simulink model "move_to_pose_R2020a1"  (R2020a)
settings: Solver=FixedStepAuto  StartTime=0.0  StopTime=inf  FixedStep=sampleTime  RelTol=1e-3
PreLoadFcn:
  | % Simulation parameters
  | load exampleMap
  | sampleTime = 0.05;
  | 
  | % Robot parameters
  | wheelRadius = 0.05;
  | robotRadius = 0.5;
  | 
  | % Lidar parameters
  | sensorOffset = [0,0];
  | scanAngles = linspace(-pi/2,pi/2,9)';
  | maxRange = 25;
undefined symbols (not defined in the file or in its folder): data_array
libraries: mobileRoboticsLib x38, robotalgslib x11, mobileRoboticsTrainingLib x11
settings Model: SimulationMode=accelerator  EnablePacing=on  PacingRate=1000  Creator=scastro  LastModifiedBy=prans
settings DataIOCC: ReturnWorkspaceOutputs=off
settings DebuggingCC: PregeneratedLibrarySubsystemCodeDiagnostic=none  ArithmeticOperatorsInVariantConditions=warning
settings SFSimCC: SimUseLocalCustomCode=off  CustomCodeUndefinedFunction=UseInterfaceOnly
settings RTWCC: RTWUseLocalCustomCode=off

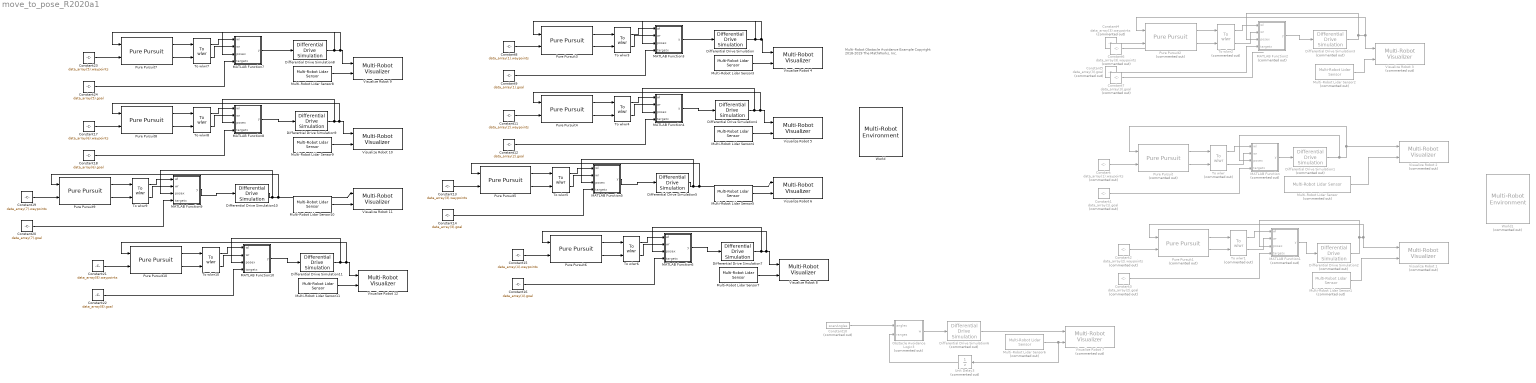
== system move_to_pose_R2020a1 ==
  note: Multi-Robot Obstacle
      | Avoidance Example
      |
      | Copyright 2018-2019 The MathWorks, Inc.
  Constant : Constant  Commented=on  Value=data_array(1).waypoints
  Constant1 : Constant  Commented=on  Value=data_array(1).goal
  Constant10 : Constant  Commented=on  Value=scanAngles
  Constant11 : Constant  Value=data_array(2).waypoints
  Constant12 : Constant  Value=data_array(2).goal
  Constant13 : Constant  Value=data_array(3).waypoints
  Constant14 : Constant  Value=data_array(3).goal
  Constant15 : Constant  Value=data_array(4).waypoints
  Constant16 : Constant  Value=data_array(4).goal
  Constant17 : Constant  Value=data_array(6).waypoints
  Constant18 : Constant  Value=data_array(6).goal
  Constant19 : Constant  Value=data_array(7).waypoints
  Constant2 : Constant  Commented=on  Value=data_array(2).waypoints
  Constant20 : Constant  Value=data_array(7).goal
  Constant21 : Constant  Value=data_array(8).waypoints
  Constant22 : Constant  Value=data_array(8).goal
  Constant23 : Constant  Value=data_array(5).waypoints
  Constant24 : Constant  Value=data_array(5).goal
  Constant3 : Constant  Commented=on  Value=data_array(2).goal
  Constant4 : Constant  Commented=on  Value=data_array(3).waypoints
  Constant5 : Constant  Commented=on  Value=data_array(3).goal
  Constant6 : Constant  Commented=on  Value=data_array(3).waypoints
  Constant7 : Constant  Commented=on  Value=data_array(3).goal
  Constant8 : Constant  Value=data_array(1).waypoints
  Constant9 : Constant  Value=data_array(1).goal
  Differential Drive Simulation : mobileRoboticsLib/Kinematic Models/Differential Drive/Differential Drive Simulation  wheelRadius=wheelRadius  wheelBase=robotRadius  initX=data_array(1).start(1)  initY=data_array(1).start(2)  initAngle=0  Ts=sampleTime
      settings: SourceProductName=Mobile Robotics Simulation Toolbox
  Differential Drive Simulation1 : mobileRoboticsLib/Kinematic Models/Differential Drive/Differential Drive Simulation  Commented=on  wheelRadius=wheelRadius  wheelBase=robotRadius  initX=data_array(1).start(1)  initY=data_array(1).start(2)  initAngle=0  Ts=sampleTime
      settings: SourceProductName=Mobile Robotics Simulation Toolbox
  Differential Drive Simulation10 : mobileRoboticsLib/Kinematic Models/Differential Drive/Differential Drive Simulation  wheelRadius=wheelRadius  wheelBase=robotRadius  initX=data_array(7).start(1)  initY=data_array(7).start(2)  initAngle=-pi/4  Ts=sampleTime
      settings: SourceProductName=Mobile Robotics Simulation Toolbox
  Differential Drive Simulation11 : mobileRoboticsLib/Kinematic Models/Differential Drive/Differential Drive Simulation  wheelRadius=wheelRadius  wheelBase=robotRadius  initX=data_array(8).start(1)  initY=data_array(8).start(2)  initAngle=-pi/4  Ts=sampleTime
      settings: SourceProductName=Mobile Robotics Simulation Toolbox
  Differential Drive Simulation2 : mobileRoboticsLib/Kinematic Models/Differential Drive/Differential Drive Simulation  Commented=on  wheelRadius=wheelRadius  wheelBase=robotRadius  initX=data_array(2).start(1)  initY=data_array(2).start(2)  initAngle=pi/2  Ts=sampleTime
      settings: SourceProductName=Mobile Robotics Simulation Toolbox
  Differential Drive Simulation3 : mobileRoboticsLib/Kinematic Models/Differential Drive/Differential Drive Simulation  Commented=on  wheelRadius=wheelRadius  wheelBase=robotRadius  initX=data_array(3).start(1)  initY=data_array(3).start(2)  initAngle=-pi/4  Ts=sampleTime
      settings: SourceProductName=Mobile Robotics Simulation Toolbox
  Differential Drive Simulation4 : mobileRoboticsLib/Kinematic Models/Differential Drive/Differential Drive Simulation  wheelRadius=wheelRadius  wheelBase=robotRadius  initX=data_array(2).start(1)  initY=data_array(2).start(2)  initAngle=pi/2  Ts=sampleTime
      settings: SourceProductName=Mobile Robotics Simulation Toolbox
  Differential Drive Simulation5 : mobileRoboticsLib/Kinematic Models/Differential Drive/Differential Drive Simulation  wheelRadius=wheelRadius  wheelBase=robotRadius  initX=data_array(3).start(1)  initY=data_array(3).start(2)  initAngle=-pi/4  Ts=sampleTime
      settings: SourceProductName=Mobile Robotics Simulation Toolbox
  Differential Drive Simulation6 : mobileRoboticsLib/Kinematic Models/Differential Drive/Differential Drive Simulation  Commented=on  wheelRadius=wheelRadius  wheelBase=robotRadius  initX=8  initY=8  initAngle=-pi/4  Ts=sampleTime
      settings: SourceProductName=Mobile Robotics Simulation Toolbox
  Differential Drive Simulation7 : mobileRoboticsLib/Kinematic Models/Differential Drive/Differential Drive Simulation  wheelRadius=wheelRadius  wheelBase=robotRadius  initX=data_array(4).start(1)  initY=data_array(4).start(2)  initAngle=-pi/4  Ts=sampleTime
      settings: SourceProductName=Mobile Robotics Simulation Toolbox
  Differential Drive Simulation8 : mobileRoboticsLib/Kinematic Models/Differential Drive/Differential Drive Simulation  wheelRadius=wheelRadius  wheelBase=robotRadius  initX=data_array(5).start(1)  initY=data_array(5).start(2)  initAngle=0  Ts=sampleTime
      settings: SourceProductName=Mobile Robotics Simulation Toolbox
  Differential Drive Simulation9 : mobileRoboticsLib/Kinematic Models/Differential Drive/Differential Drive Simulation  wheelRadius=wheelRadius  wheelBase=robotRadius  initX=data_array(6).start(1)  initY=data_array(6).start(2)  initAngle=pi/2  Ts=sampleTime
      settings: SourceProductName=Mobile Robotics Simulation Toolbox
  MATLAB Function : MATLAB Function  Commented=on  TreatAsAtomicUnit=on
  MATLAB Function1 : MATLAB Function  Commented=on  TreatAsAtomicUnit=on
  MATLAB Function10 : MATLAB Function  TreatAsAtomicUnit=on
  MATLAB Function2 : MATLAB Function  Commented=on  TreatAsAtomicUnit=on
  MATLAB Function3 : MATLAB Function  TreatAsAtomicUnit=on
  MATLAB Function4 : MATLAB Function  TreatAsAtomicUnit=on
  MATLAB Function5 : MATLAB Function  TreatAsAtomicUnit=on
  MATLAB Function6 : MATLAB Function  TreatAsAtomicUnit=on
  MATLAB Function7 : MATLAB Function  TreatAsAtomicUnit=on
  MATLAB Function8 : MATLAB Function  TreatAsAtomicUnit=on
  MATLAB Function9 : MATLAB Function  TreatAsAtomicUnit=on
  Multi-Robot Lidar Sensor : mobileRoboticsLib/Environments/Multi-Robot Lidar Sensor  Commented=on  robotIdx=1  mapName=map  sensorOffset=sensorOffset  scanAngles=scanAngles  maxRange=maxRange
      settings: SourceProductName=Mobile Robotics Simulation Toolbox
  Multi-Robot Lidar Sensor1 : mobileRoboticsLib/Environments/Multi-Robot Lidar Sensor  Commented=on  robotIdx=2  mapName=map  sensorOffset=sensorOffset  scanAngles=scanAngles  maxRange=maxRange
      settings: SourceProductName=Mobile Robotics Simulation Toolbox
  Multi-Robot Lidar Sensor10 : mobileRoboticsLib/Environments/Multi-Robot Lidar Sensor  robotIdx=7  mapName=map  sensorOffset=sensorOffset  scanAngles=scanAngles  maxRange=maxRange
      settings: SourceProductName=Mobile Robotics Simulation Toolbox
  Multi-Robot Lidar Sensor11 : mobileRoboticsLib/Environments/Multi-Robot Lidar Sensor  robotIdx=8  mapName=map  sensorOffset=sensorOffset  scanAngles=scanAngles  maxRange=maxRange
      settings: SourceProductName=Mobile Robotics Simulation Toolbox
  Multi-Robot Lidar Sensor2 : mobileRoboticsLib/Environments/Multi-Robot Lidar Sensor  Commented=on  robotIdx=3  mapName=map  sensorOffset=sensorOffset  scanAngles=scanAngles  maxRange=maxRange
      settings: SourceProductName=Mobile Robotics Simulation Toolbox
  Multi-Robot Lidar Sensor3 : mobileRoboticsLib/Environments/Multi-Robot Lidar Sensor  robotIdx=1  mapName=map  sensorOffset=sensorOffset  scanAngles=scanAngles  maxRange=maxRange
      settings: SourceProductName=Mobile Robotics Simulation Toolbox
  Multi-Robot Lidar Sensor4 : mobileRoboticsLib/Environments/Multi-Robot Lidar Sensor  robotIdx=2  mapName=map  sensorOffset=sensorOffset  scanAngles=scanAngles  maxRange=maxRange
      settings: SourceProductName=Mobile Robotics Simulation Toolbox
  Multi-Robot Lidar Sensor5 : mobileRoboticsLib/Environments/Multi-Robot Lidar Sensor  robotIdx=3  mapName=map  sensorOffset=sensorOffset  scanAngles=scanAngles  maxRange=maxRange
      settings: SourceProductName=Mobile Robotics Simulation Toolbox
  Multi-Robot Lidar Sensor6 : mobileRoboticsLib/Environments/Multi-Robot Lidar Sensor  Commented=on  robotIdx=4  mapName=map  sensorOffset=sensorOffset  scanAngles=scanAngles  maxRange=maxRange
      settings: SourceProductName=Mobile Robotics Simulation Toolbox
  Multi-Robot Lidar Sensor7 : mobileRoboticsLib/Environments/Multi-Robot Lidar Sensor  robotIdx=4  mapName=map  sensorOffset=sensorOffset  scanAngles=scanAngles  maxRange=maxRange
      settings: SourceProductName=Mobile Robotics Simulation Toolbox
  Multi-Robot Lidar Sensor8 : mobileRoboticsLib/Environments/Multi-Robot Lidar Sensor  robotIdx=5  mapName=map  sensorOffset=sensorOffset  scanAngles=scanAngles  maxRange=maxRange
      settings: SourceProductName=Mobile Robotics Simulation Toolbox
  Multi-Robot Lidar Sensor9 : mobileRoboticsLib/Environments/Multi-Robot Lidar Sensor  robotIdx=6  mapName=map  sensorOffset=sensorOffset  scanAngles=scanAngles  maxRange=maxRange
      settings: SourceProductName=Mobile Robotics Simulation Toolbox
  Obstacle Avoidance Logic3 : Stateflow chart  Commented=on  TreatAsAtomicUnit=on
  Pure Pursuit : robotalgslib/Pure Pursuit  Commented=on  DesiredLinearVelocity=0.1  MaxAngularVelocity=1  LookaheadDistance=1  TargetDirPort=off  SimulateUsing=Code generation
  Pure Pursuit1 : robotalgslib/Pure Pursuit  Commented=on  DesiredLinearVelocity=0.1  MaxAngularVelocity=1  LookaheadDistance=1  TargetDirPort=off  SimulateUsing=Code generation
  Pure Pursuit{3..10} (8 alike) : robotalgslib/Pure Pursuit  DesiredLinearVelocity=0.1  MaxAngularVelocity=1  LookaheadDistance=1  TargetDirPort=off  SimulateUsing=Code generation
  Pure Pursuit2 : robotalgslib/Pure Pursuit  Commented=on  DesiredLinearVelocity=0.1  MaxAngularVelocity=1  LookaheadDistance=1  TargetDirPort=off  SimulateUsing=Code generation
  To wlwr : mobileRoboticsTrainingLib/To wlwr  Commented=on  axleLength=0.1  wheelR=0.05
  To wlwr1 : mobileRoboticsTrainingLib/To wlwr  Commented=on  axleLength=0.1  wheelR=0.05
  To wlwr{3..10} (8 alike) : mobileRoboticsTrainingLib/To wlwr  axleLength=0.1  wheelR=0.05
  To wlwr2 : mobileRoboticsTrainingLib/To wlwr  Commented=on  axleLength=0.1  wheelR=0.05
  Unit Delay3 : UnitDelay  Commented=on  SampleTime=-1  HasFrameUpgradeWarning=on
  Visualize Robot 1 : mobileRoboticsLib/Environments/Multi-Robot Visualizer  Commented=on  idx=2  radius=robotRadius  robotColor=[0 0 1]  showTraj=off  hasLidar=on  sensorOffset=sensorOffset  scanAngles=scanAngles  maxNumScans=0  hasObjDetector=off  objDetectorOffset=[0 0]  objDetectorAngle=0  objDetectorFOV=pi/2  objDetectorMaxRange=5  hasRobotDetector=off  robotDetectorOffset=[0,0]  robotDetectorAngle=0  robotDetectorFOV=pi/3  robotDetectorMaxRange=5  robotDetectorNumDetections=0
      settings: SourceProductName=Mobile Robotics Simulation Toolbox
  Visualize Robot 10 : mobileRoboticsLib/Environments/Multi-Robot Visualizer  idx=6  radius=robotRadius  robotColor=[1 1 0]  showTraj=on  hasLidar=on  sensorOffset=sensorOffset  scanAngles=scanAngles  maxNumScans=0  hasObjDetector=off  objDetectorOffset=[0 0]  objDetectorAngle=0  objDetectorFOV=pi/2  objDetectorMaxRange=5  hasRobotDetector=off  robotDetectorOffset=[0,0]  robotDetectorAngle=0  robotDetectorFOV=pi/3  robotDetectorMaxRange=5  robotDetectorNumDetections=0
      settings: SourceProductName=Mobile Robotics Simulation Toolbox
  Visualize Robot 11 : mobileRoboticsLib/Environments/Multi-Robot Visualizer  idx=7  radius=robotRadius  robotColor=[1 1 1]  showTraj=on  hasLidar=on  sensorOffset=sensorOffset  scanAngles=scanAngles  maxNumScans=0  hasObjDetector=off  objDetectorOffset=[0 0]  objDetectorAngle=0  objDetectorFOV=pi/2  objDetectorMaxRange=5  hasRobotDetector=off  robotDetectorOffset=[0,0]  robotDetectorAngle=0  robotDetectorFOV=pi/3  robotDetectorMaxRange=5  robotDetectorNumDetections=0
      settings: SourceProductName=Mobile Robotics Simulation Toolbox
  Visualize Robot 12 : mobileRoboticsLib/Environments/Multi-Robot Visualizer  idx=8  radius=robotRadius  robotColor=[0 0 0]  showTraj=on  hasLidar=on  sensorOffset=sensorOffset  scanAngles=scanAngles  maxNumScans=0  hasObjDetector=off  objDetectorOffset=[0 0]  objDetectorAngle=0  objDetectorFOV=pi/2  objDetectorMaxRange=5  hasRobotDetector=off  robotDetectorOffset=[0,0]  robotDetectorAngle=0  robotDetectorFOV=pi/3  robotDetectorMaxRange=5  robotDetectorNumDetections=0
      settings: SourceProductName=Mobile Robotics Simulation Toolbox
  Visualize Robot 2 : mobileRoboticsLib/Environments/Multi-Robot Visualizer  Commented=on  idx=1  radius=robotRadius  robotColor=[1 0 0]  showTraj=off  hasLidar=on  sensorOffset=sensorOffset  scanAngles=scanAngles  maxNumScans=0  hasObjDetector=off  objDetectorOffset=[0,0]  objDetectorAngle=0  objDetectorFOV=pi/2  objDetectorMaxRange=5  hasRobotDetector=off  robotDetectorOffset=sensorOffset  robotDetectorAngle=[pi/2 -pi/2]  robotDetectorFOV=pi  robotDetectorMaxRange=25  robotDetectorNumDetections=0
      link override Goto_ObjDetector: GotoTag=slMultiRobotEnv_ObjDet_2
      link override Goto_Pose: GotoTag=slMultiRobotEnv_Pose_2
      link override Goto_Ranges: GotoTag=slMultiRobotEnv_Ranges_2
      link override Goto_RobotDetector: GotoTag=slMultiRobotEnv_RobotDet_2
      link override Goto_Visuals: GotoTag=slMultiRobotEnv_Visuals_2
      settings: SourceProductName=Mobile Robotics Simulation Toolbox
  Visualize Robot 3 : mobileRoboticsLib/Environments/Multi-Robot Visualizer  Commented=on  idx=3  radius=robotRadius  robotColor=[0 0 1]  showTraj=off  hasLidar=on  sensorOffset=sensorOffset  scanAngles=scanAngles  maxNumScans=0  hasObjDetector=off  objDetectorOffset=[0 0]  objDetectorAngle=0  objDetectorFOV=pi/2  objDetectorMaxRange=5  hasRobotDetector=off  robotDetectorOffset=[0,0]  robotDetectorAngle=0  robotDetectorFOV=pi/3  robotDetectorMaxRange=5  robotDetectorNumDetections=0
      settings: SourceProductName=Mobile Robotics Simulation Toolbox
  Visualize Robot 4 : mobileRoboticsLib/Environments/Multi-Robot Visualizer  idx=1  radius=robotRadius  robotColor=[0 0 1]  showTraj=on  hasLidar=on  sensorOffset=sensorOffset  scanAngles=scanAngles  maxNumScans=0  hasObjDetector=off  objDetectorOffset=[0,0]  objDetectorAngle=0  objDetectorFOV=pi/2  objDetectorMaxRange=5  hasRobotDetector=off  robotDetectorOffset=[0,0]  robotDetectorAngle=0  robotDetectorFOV=pi/3  robotDetectorMaxRange=5  robotDetectorNumDetections=0
      settings: SourceProductName=Mobile Robotics Simulation Toolbox
  Visualize Robot 5 : mobileRoboticsLib/Environments/Multi-Robot Visualizer  idx=2  radius=robotRadius  robotColor=[0 1 0]  showTraj=on  hasLidar=on  sensorOffset=sensorOffset  scanAngles=scanAngles  maxNumScans=0  hasObjDetector=off  objDetectorOffset=[0 0]  objDetectorAngle=0  objDetectorFOV=pi/2  objDetectorMaxRange=5  hasRobotDetector=off  robotDetectorOffset=[0,0]  robotDetectorAngle=0  robotDetectorFOV=pi/3  robotDetectorMaxRange=5  robotDetectorNumDetections=0
      settings: SourceProductName=Mobile Robotics Simulation Toolbox
  Visualize Robot 6 : mobileRoboticsLib/Environments/Multi-Robot Visualizer  idx=3  radius=robotRadius  robotColor=[0 1 1]  showTraj=on  hasLidar=on  sensorOffset=sensorOffset  scanAngles=scanAngles  maxNumScans=0  hasObjDetector=off  objDetectorOffset=[0 0]  objDetectorAngle=0  objDetectorFOV=pi/2  objDetectorMaxRange=5  hasRobotDetector=off  robotDetectorOffset=[0,0]  robotDetectorAngle=0  robotDetectorFOV=pi/3  robotDetectorMaxRange=5  robotDetectorNumDetections=0
      settings: SourceProductName=Mobile Robotics Simulation Toolbox
  Visualize Robot 7 : mobileRoboticsLib/Environments/Multi-Robot Visualizer  Commented=on  idx=4  radius=robotRadius  robotColor=[0 0 1]  showTraj=off  hasLidar=on  sensorOffset=sensorOffset  scanAngles=scanAngles  maxNumScans=0  hasObjDetector=off  objDetectorOffset=[0 0]  objDetectorAngle=0  objDetectorFOV=pi/2  objDetectorMaxRange=5  hasRobotDetector=off  robotDetectorOffset=[0,0]  robotDetectorAngle=0  robotDetectorFOV=pi/3  robotDetectorMaxRange=5  robotDetectorNumDetections=0
      settings: SourceProductName=Mobile Robotics Simulation Toolbox
  Visualize Robot 8 : mobileRoboticsLib/Environments/Multi-Robot Visualizer  idx=4  radius=robotRadius  robotColor=[1 0 0]  showTraj=on  hasLidar=on  sensorOffset=sensorOffset  scanAngles=scanAngles  maxNumScans=0  hasObjDetector=off  objDetectorOffset=[0 0]  objDetectorAngle=0  objDetectorFOV=pi/2  objDetectorMaxRange=5  hasRobotDetector=off  robotDetectorOffset=[0,0]  robotDetectorAngle=0  robotDetectorFOV=pi/3  robotDetectorMaxRange=5  robotDetectorNumDetections=0
      settings: SourceProductName=Mobile Robotics Simulation Toolbox
  Visualize Robot 9 : mobileRoboticsLib/Environments/Multi-Robot Visualizer  idx=5  radius=robotRadius  robotColor=[1 0 1]  showTraj=on  hasLidar=on  sensorOffset=sensorOffset  scanAngles=scanAngles  maxNumScans=0  hasObjDetector=off  objDetectorOffset=[0,0]  objDetectorAngle=0  objDetectorFOV=pi/2  objDetectorMaxRange=5  hasRobotDetector=off  robotDetectorOffset=[0,0]  robotDetectorAngle=0  robotDetectorFOV=pi/3  robotDetectorMaxRange=5  robotDetectorNumDetections=0
      settings: SourceProductName=Mobile Robotics Simulation Toolbox
  World : mobileRoboticsLib/Environments/Multi-Robot Environment  numRobots=8  mapName=map  showWaypoints=off  showObjects=off  objectColors=[1 0 0;0 1 0;0 0 1]  objectMarkers='s'  showRobotIds=on  plotSensorLines=on
      settings: SourceProductName=Mobile Robotics Simulation Toolbox
  World1 : mobileRoboticsLib/Environments/Multi-Robot Environment  Commented=on  numRobots=1  mapName=map  showWaypoints=off  showObjects=off  objectColors=[1 0 0;0 1 0;0 0 1]  objectMarkers='s'  showRobotIds=on  plotSensorLines=on
      settings: SourceProductName=Mobile Robotics Simulation Toolbox
  wires:
  Multi-Robot Lidar Sensor1/1 -> Visualize Robot 1/2
  Multi-Robot Lidar Sensor2/1 -> Visualize Robot 3/2
  MATLAB Function1/1(y) -> Differential Drive Simulation2/1
  To wlwr1/1 -> MATLAB Function1/1(wl)
  Differential Drive Simulation2/1 -> MATLAB Function1/3(posex), Visualize Robot 1/1, Pure Pursuit1/1
  To wlwr1/2 -> MATLAB Function1/2(wr)
  Constant2/1 -> Pure Pursuit1/2
  Pure Pursuit1/2 -> To wlwr1/2
  Pure Pursuit1/1 -> To wlwr1/1
  Constant3/1 -> MATLAB Function1/4(targetx)
  Constant4/1 -> Pure Pursuit2/2
  To wlwr2/1 -> MATLAB Function2/1(wl)
  Constant5/1 -> MATLAB Function2/4(targetx)
  To wlwr2/2 -> MATLAB Function2/2(wr)
  Pure Pursuit2/1 -> To wlwr2/1
  Differential Drive Simulation3/1 -> Pure Pursuit2/1, Visualize Robot 3/1, MATLAB Function2/3(posex)
  MATLAB Function2/1(y) -> Differential Drive Simulation3/1
  Pure Pursuit2/2 -> To wlwr2/2
  To wlwr/2 -> MATLAB Function/2(wr)
  Constant/1 -> Pure Pursuit/2
  MATLAB Function/1(y) -> Differential Drive Simulation1/1
  To wlwr/1 -> MATLAB Function/1(wl)
  Multi-Robot Lidar Sensor/1 -> Visualize Robot 2/2
  Pure Pursuit/2 -> To wlwr/2
  Pure Pursuit/1 -> To wlwr/1
  Differential Drive Simulation1/1 -> MATLAB Function/3(posex), Pure Pursuit/1, Visualize Robot 2/1
  Constant1/1 -> MATLAB Function/4(targetx)
  Differential Drive Simulation6/1 -> Visualize Robot 7/1
  Multi-Robot Lidar Sensor3/1 -> Visualize Robot 4/2
  To wlwr3/1 -> MATLAB Function3/1(wl)
  Differential Drive Simulation/1 -> MATLAB Function3/3(posex), Pure Pursuit3/1, Visualize Robot 4/1
  Pure Pursuit3/1 -> To wlwr3/1
  Pure Pursuit3/2 -> To wlwr3/2
  Constant6/1 -> ?
  Constant7/1 -> ?
  Constant8/1 -> Pure Pursuit3/2
  Constant9/1 -> MATLAB Function3/4(targetx)
  MATLAB Function3/1(y) -> Differential Drive Simulation/1
  To wlwr3/2 -> MATLAB Function3/2(wr)
  Obstacle Avoidance Logic3/1(w) -> Differential Drive Simulation6/1
  Unit Delay3/1 -> Obstacle Avoidance Logic3/2(ranges)
  Constant10/1 -> Obstacle Avoidance Logic3/1(angles)
  Multi-Robot Lidar Sensor4/1 -> Visualize Robot 5/2
  Multi-Robot Lidar Sensor5/1 -> Visualize Robot 6/2
  Multi-Robot Lidar Sensor6/1 -> Unit Delay3/1, Visualize Robot 7/2
  Pure Pursuit4/1 -> To wlwr4/1
  To wlwr4/2 -> MATLAB Function4/2(wr)
  Constant12/1 -> MATLAB Function4/4(targetx)
  Pure Pursuit4/2 -> To wlwr4/2
  Constant11/1 -> Pure Pursuit4/2
  To wlwr4/1 -> MATLAB Function4/1(wl)
  Differential Drive Simulation4/1 -> MATLAB Function4/3(posex), Pure Pursuit4/1, Visualize Robot 5/1
  MATLAB Function4/1(y) -> Differential Drive Simulation4/1
  To wlwr5/2 -> MATLAB Function5/2(wr)
  Differential Drive Simulation5/1 -> MATLAB Function5/3(posex), Pure Pursuit5/1, Visualize Robot 6/1
  Constant13/1 -> Pure Pursuit5/2
  Pure Pursuit5/2 -> To wlwr5/2
  Pure Pursuit5/1 -> To wlwr5/1
  MATLAB Function5/1(y) -> Differential Drive Simulation5/1
  Constant14/1 -> MATLAB Function5/4(targetx)
  To wlwr5/1 -> MATLAB Function5/1(wl)
  Multi-Robot Lidar Sensor7/1 -> Visualize Robot 8/2
  To wlwr6/2 -> MATLAB Function6/2(wr)
  Differential Drive Simulation7/1 -> MATLAB Function6/3(posex), Pure Pursuit6/1, Visualize Robot 8/1
  Constant15/1 -> Pure Pursuit6/2
  Pure Pursuit6/2 -> To wlwr6/2
  Pure Pursuit6/1 -> To wlwr6/1
  MATLAB Function6/1(y) -> Differential Drive Simulation7/1
  Constant16/1 -> MATLAB Function6/4(targetx)
  To wlwr6/1 -> MATLAB Function6/1(wl)
  MATLAB Function9/1(y) -> Differential Drive Simulation10/1
  Multi-Robot Lidar Sensor11/1 -> Visualize Robot 12/2
  MATLAB Function8/1(y) -> Differential Drive Simulation9/1
  Pure Pursuit8/1 -> To wlwr8/1
  Constant22/1 -> MATLAB Function10/4(targetx)
  To wlwr8/2 -> MATLAB Function8/2(wr)
  Pure Pursuit7/1 -> To wlwr7/1
  Constant19/1 -> Pure Pursuit9/2
  To wlwr7/2 -> MATLAB Function7/2(wr)
  Constant24/1 -> MATLAB Function7/4(targetx)
  Constant23/1 -> Pure Pursuit7/2
  Constant20/1 -> MATLAB Function9/4(targetx)
  To wlwr9/1 -> MATLAB Function9/1(wl)
  Pure Pursuit10/1 -> To wlwr10/1
  To wlwr10/2 -> MATLAB Function10/2(wr)
  To wlwr10/1 -> MATLAB Function10/1(wl)
  Pure Pursuit7/2 -> To wlwr7/2
  Pure Pursuit10/2 -> To wlwr10/2
  MATLAB Function10/1(y) -> Differential Drive Simulation11/1
  Differential Drive Simulation8/1 -> MATLAB Function7/3(posex), Pure Pursuit7/1, Visualize Robot 9/1
  Differential Drive Simulation10/1 -> MATLAB Function9/3(posex), Pure Pursuit9/1, Visualize Robot 11/1
  Differential Drive Simulation9/1 -> MATLAB Function8/3(posex), Pure Pursuit8/1, Visualize Robot 10/1
  To wlwr7/1 -> MATLAB Function7/1(wl)
  Pure Pursuit9/2 -> To wlwr9/2
  Multi-Robot Lidar Sensor10/1 -> Visualize Robot 11/2
  Multi-Robot Lidar Sensor9/1 -> Visualize Robot 10/2
  Multi-Robot Lidar Sensor8/1 -> Visualize Robot 9/2
  Differential Drive Simulation11/1 -> MATLAB Function10/3(posex), Pure Pursuit10/1, Visualize Robot 12/1
  Pure Pursuit8/2 -> To wlwr8/2
  MATLAB Function7/1(y) -> Differential Drive Simulation8/1
  Constant21/1 -> Pure Pursuit10/2
  Constant17/1 -> Pure Pursuit8/2
  To wlwr8/1 -> MATLAB Function8/1(wl)
  To wlwr9/2 -> MATLAB Function9/2(wr)
  Constant18/1 -> MATLAB Function8/4(targetx)
  Pure Pursuit9/1 -> To wlwr9/1

== stateflow chart move_to_pose_R2020a1/Obstacle Avoidance Logic3 ==
  state MainState [parallel]
    en,du:
    validIdx = ~isnan(ranges);
    validRanges = ranges(validIdx);
    validAngles = angles(validIdx);
    settings: executionOrder=1
    state Turn
      en,du:
      avgAngle = mean(validAngles./validRanges);
      state Left
        en, du:
        w = [0;12.5];
      state Right
        en, du:
        w = [12.5;0];
      (default) -> (junction 39)
      (junction 39) -> Left [order 1] : [avgAngle < 0]
      (junction 39) -> (junction 43) [order 2]
      Left -> Right : [after(1,sec) && ...
          | avgAngle > 0]
      Right -> Left : [after(1,sec) && ...
          | avgAngle < 0]
      (junction 43) -> Right
    state GoStraight
      en:
      w = [25; 25];
    (default) -> GoStraight
    GoStraight -> Turn : [any(validRanges<=1)]
    Turn -> GoStraight : [all(validRanges>1)]
  data: angles input; w output; ranges input; validRanges local size=numel(scanAngles); validIdx local; validAngles local size=numel(scanAngles); avgAngle local

== matlab function move_to_pose_R2020a1/MATLAB Function6 ==
  data: wl input; y output; wr input; posex input; targetx input
function y = fcn(wl, wr, posex, targetx)
    if (abs(posex(1) - targetx(1)) < 0.02 && abs(posex(2) - targetx(2)) < 0.02)
        y = [0 0];
    else
        y = [wl, wr];
    end
end

== matlab function move_to_pose_R2020a1/MATLAB Function10 ==
  data: wl input; y output; wr input; posex input; targetx input
function y = fcn(wl, wr, posex, targetx)
    if (abs(posex(1) - targetx(1)) < 0.02 && abs(posex(2) - targetx(2)) < 0.02)
        y = [0 0];
    else
        y = [wl, wr];
    end
end

== matlab function move_to_pose_R2020a1/MATLAB Function7 ==
  data: wl input; y output; wr input; posex input; targetx input
function y = fcn(wl, wr, posex, targetx)
    if (abs(posex(1) - targetx(1)) < 0.02 && abs(posex(2) - targetx(2)) < 0.02)
        y = [0 0];
    else
        y = [wl, wr];
    end
end

== matlab function move_to_pose_R2020a1/MATLAB Function8 ==
  data: wl input; y output; wr input; posex input; targetx input
function y = fcn(wl, wr, posex, targetx)
    if (abs(posex(1) - targetx(1)) < 0.02 && abs(posex(2) - targetx(2)) < 0.02)
        y = [0 0];
    else
        y = [wl, wr];
    end
end

== matlab function move_to_pose_R2020a1/MATLAB Function9 ==
  data: wl input; y output; wr input; posex input; targetx input
function y = fcn(wl, wr, posex, targetx)
    if (abs(posex(1) - targetx(1)) < 0.02 && abs(posex(2) - targetx(2)) < 0.02)
        y = [0 0];
    else
        y = [wl, wr];
    end
end

== matlab function move_to_pose_R2020a1/MATLAB Function1 ==
  data: wl input; y output; wr input; posex input; targetx input
function y = fcn(wl, wr, posex, targetx)
    if (abs(posex(1) - targetx(1)) < 0.02 && abs(posex(2) - targetx(2)) < 0.02)
        y = [0 0];
    else
        y = [wl, wr];
    end
end

== matlab function move_to_pose_R2020a1/MATLAB Function3 ==
  data: wl input; y output; wr input; posex input; targetx input
function y = fcn(wl, wr, posex, targetx)
    if (abs(posex(1) - targetx(1)) < 0.02 && abs(posex(2) - targetx(2)) < 0.02)
        y = [0 0];
    else
        y = [wl, wr];
    end
end

== matlab function move_to_pose_R2020a1/MATLAB Function2 ==
  data: wl input; y output; wr input; posex input; targetx input
function y = fcn(wl, wr, posex, targetx)
    if (abs(posex(1) - targetx(1)) < 0.02 && abs(posex(2) - targetx(2)) < 0.02)
        y = [0 0];
    else
        y = [wl, wr];
    end
end

== matlab function move_to_pose_R2020a1/MATLAB Function4 ==
  data: wl input; y output; wr input; posex input; targetx input
function y = fcn(wl, wr, posex, targetx)
    if (abs(posex(1) - targetx(1)) < 0.02 && abs(posex(2) - targetx(2)) < 0.02)
        y = [0 0];
    else
        y = [wl, wr];
    end
end

== matlab function move_to_pose_R2020a1/MATLAB Function ==
  data: wl input; y output; wr input; posex input; targetx input
function y = fcn(wl, wr, posex, targetx)
    if (abs(posex(1) - targetx(1)) < 0.02 && abs(posex(2) - targetx(2)) < 0.02)
        y = [0 0];
    else
        y = [wl, wr];
    end
end

== matlab function move_to_pose_R2020a1/MATLAB Function5 ==
  data: wl input; y output; wr input; posex input; targetx input
function y = fcn(wl, wr, posex, targetx)
    if (abs(posex(1) - targetx(1)) < 0.02 && abs(posex(2) - targetx(2)) < 0.02)
        y = [0 0];
    else
        y = [wl, wr];
    end
end
